simulink model "Small_system"  (R2025b)
settings: Solver=ode8  StartTime=0.0  StopTime=105  FixedStep=1  RelTol=1e-3
model workspace (MAT data in the model file):
  Sig = Simulink.Signal
  Sig.Dimensions = -1
  Sig.DimensionsMode = 'auto'
  Sig.Complexity = 'auto'
  Sig.SampleTime = -1
  Sig.SamplingMode = 'auto'
  Sig.DataType = 'auto'
settings Model: Creator=Soere  LastModifiedBy=klump
settings DebuggingCC: UnderSpecifiedDimensionMsg=warning

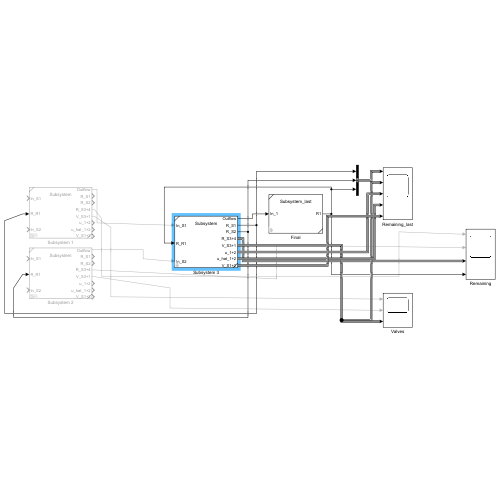
[thumbnail: Simulink's stored preview of the top-level diagram]
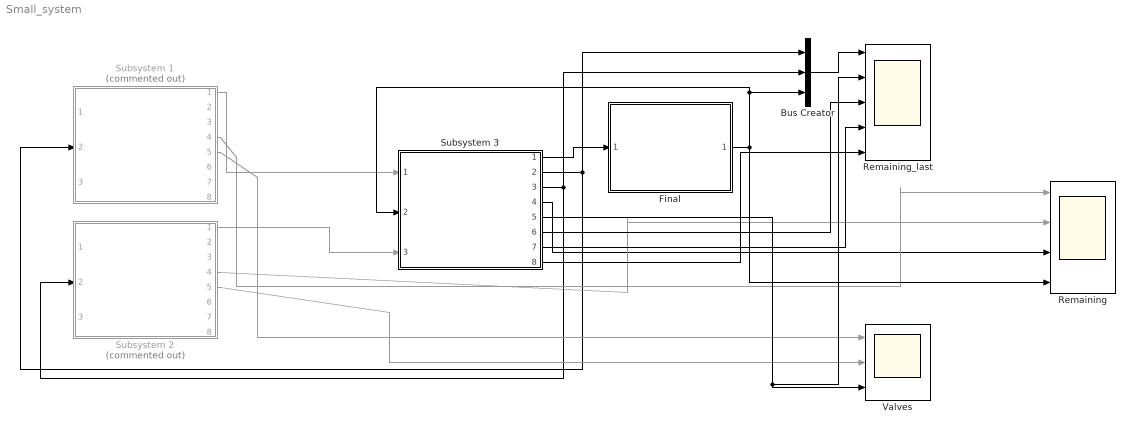
== system Small_system ==
  Bus Creator : BusCreator  Inputs=3
  Final : Subsystem  ReferencedSubsystem=Subsystem_last  Diameter=23.3  Max_cap_1=510-150  Waterlevel_1=158-150  proces=0
  Remaining : Scope  NumInputPorts=4
      settings: ActiveDisplayString=3  ActiveDisplayYMinimum=-22.646288209607036  ActiveDisplayYMaximum=313.353711790393  DataLoggingVariableName=ScopeData4
  Remaining_last : Scope  NumInputPorts=5
      settings: ActiveDisplayYMinimum=-1  ActiveDisplayYMaximum=15.5  YLabel=Remaining capacity (liters)  DataLoggingVariableName=ScopeData19
  Subsystem 1 : Subsystem  Commented=on  ReferencedSubsystem=Subsystem  Waterlevel_1=0  Height=1  Max_cap_1=300  Diameter=24.5  K=7.77*1e-5  A=0.0117  B=0.1252  Duration_S1=10*60  Flowrate_S1=1  BurstStart=1  BurstFlow=1  BurstDur=1  RainSwitch_S1=off  Waterlevel_2=0  Height_2=1  Max_cap_2=300  Diameter_2=24.5  K_2=7.77*1e-5  A_2=0.0117  B_2=0.1252  Duration_S2=9*60  Flowrate_S2=1  BurstStart_2=1  BurstFlow_2=1  BurstDur_2=1  RainSwitch_S2=off  DelayLength=10
  Subsystem 2 : Subsystem  Commented=on  ReferencedSubsystem=Subsystem  Waterlevel_1=0  Height=1  Max_cap_1=300  Diameter=24.5  K=7.77*1e-5  A=0.0117  B=0.1252  Duration_S1=10*60  Flowrate_S1=1  BurstStart=1  BurstFlow=1  BurstDur=1  RainSwitch_S1=off  Waterlevel_2=0  Height_2=1  Max_cap_2=300  Diameter_2=24.5  K_2=7.77*1e-5  A_2=0.0117  B_2=0.1252  Duration_S2=9*60  Flowrate_S2=1  BurstStart_2=1  BurstFlow_2=1  BurstDur_2=1  RainSwitch_S2=off  DelayLength=10
  Subsystem 3 : Subsystem  ReferencedSubsystem=Subsystem  Waterlevel_1=(703-150)*1  Height=1  Max_cap_1=703-150  Diameter=24.5  K=7.77*1e-5  A=0.0117  B=0.1252  Duration_S1=60*8  Flowrate_S1=5  BurstStart=60*3  BurstFlow=10  BurstDur=60*2  RainSwitch_S1=off  Waterlevel_2=539-150  Height_2=1  Max_cap_2=695-150  Diameter_2=23.3  K_2=7.32*1e-5  A_2=0.0118  B_2=0.1206  Duration_S2=60*8  Flowrate_S2=5  BurstStart_2=1  BurstFlow_2=1  BurstDur_2=1  RainSwitch_S2=off  DelayLength=0
  Valves : Scope  NumInputPorts=3
      settings: ActiveDisplayString=3  ActiveDisplayYMinimum=-0.1  ActiveDisplayYMaximum=1.1  DataLoggingVariableName=ScopeData8
  wires:
  Subsystem 1/1 -> Subsystem 3/1
  Subsystem 2/1 -> Subsystem 3/3
  Subsystem 3/2 -> Subsystem 1/2, Bus Creator/1
  Subsystem 3/3 -> Subsystem 2/2, Bus Creator/2
  Subsystem 3/4 -> Remaining/3
  Subsystem 1/4 -> Remaining/1
  Subsystem 2/4 -> Remaining/2
  Subsystem 2/5 -> Valves/2
  Subsystem 1/5 -> Valves/1
  Subsystem 3/5 -> Valves/3, Remaining_last/2
  Subsystem 3/1 -> Final/1
  Final/1 -> Remaining/4, Bus Creator/3, Subsystem 3/2
  Bus Creator/1 -> Remaining_last/1
  Subsystem 3/6 -> Remaining_last/3
  Subsystem 3/7 -> Remaining_last/4
  Subsystem 3/8 -> Remaining_last/5
